simulink model "distance_tracking_slides"  (R2018b)
settings: Solver=ode8  StartTime=0.0  StopTime=20  FixedStep=0.02  RelTol=1e-3
InitFcn:
  | w = 1
  | CA = 1
  | invCB = 1
  | Ka = 1
  | Kv = 1
  | Kd = 1
  | max_accel = 1
settings Model: Creator=suvo.ganguli  LastModifiedBy=suvo.ganguli

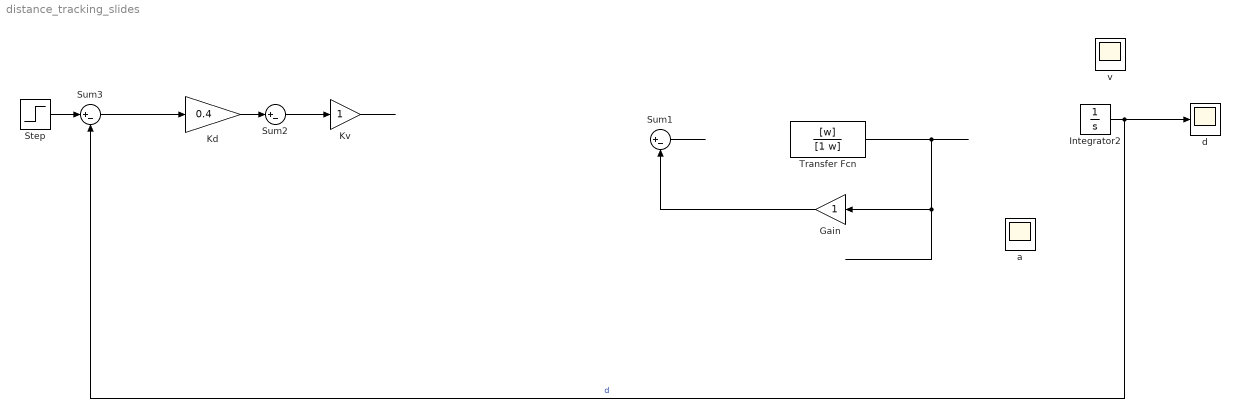
== system distance_tracking_slides ==
  Gain : Gain
  Integrator2 : Integrator
  Kd : Gain  Gain=0.4
  Kv : Gain
  Step : Step  SampleTime=0
  Sum1 : Sum  Inputs=|+-
  Sum2 : Sum  Inputs=|+-
  Sum3 : Sum  Inputs=|+-
  Transfer Fcn : TransferFcn  Numerator=[w]  Denominator=[1 w]
  a : Scope
  d : Scope
  v : Scope
  wires:
  Integrator2/1 -> d/1, Sum3/2  "d"
  Sum1/1 -> ?
  Transfer Fcn/1 -> Gain/1
  ? -> ?
  ? -> Sum1/1
  Sum2/1 -> Kv/1
  Step/1 -> Sum3/1
  Kd/1 -> Sum2/1
  Sum3/1 -> Kd/1
  Kv/1 -> ?
  ? -> Transfer Fcn/1  "j"
  Gain/1 -> Sum1/2
